simulink model "Single_Phase_Dual_converter_22UEE051"  (R2023b)
settings: Solver=VariableStepAuto  StartTime=0.0  StopTime=0.1  RelTol=1e-3
libraries: spsThyristorLib x8, spsVoltageMeasurementLib x5, spsSeriesRLCBranchLib x3, spsACVoltageSourceLib x2, spspowerguiLib x1
settings Model: Creator=prita  LastModifiedBy=SWARUP
settings DebuggingCC: UnconnectedInputMsg=warning  UnconnectedOutputMsg=warning  UnconnectedLineMsg=warning
settings ModelReferenceCC: EnableRefExpFcnMdlSchedulingChecks=on
settings RTWCC: DLArmComputeVersion=19.05

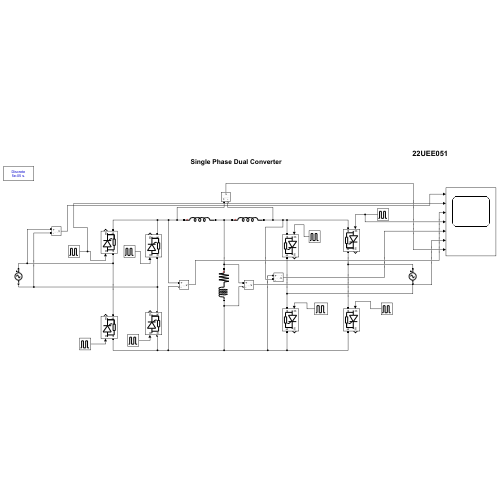
[thumbnail: Simulink's stored preview of the top-level diagram]
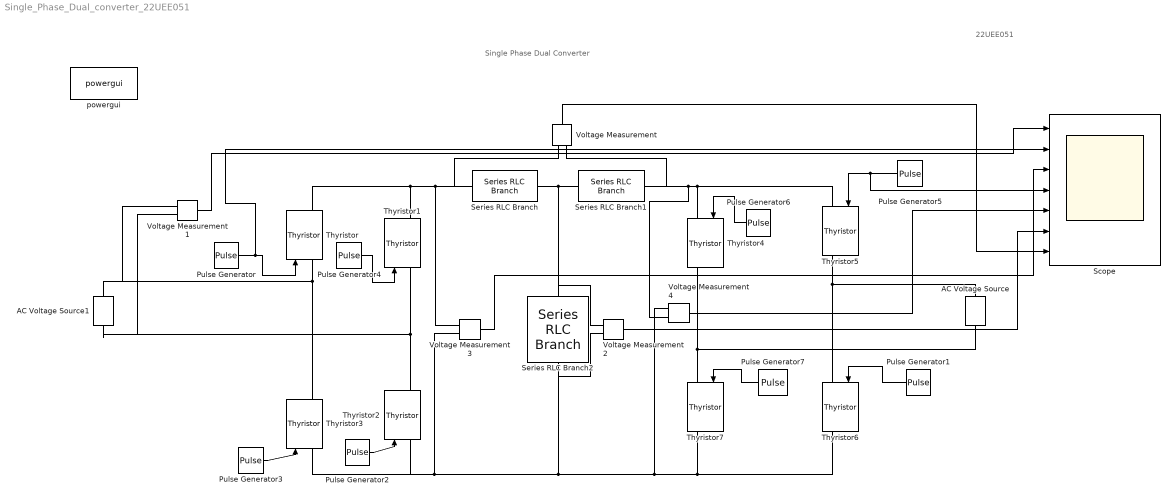
== system Single_Phase_Dual_converter_22UEE051 ==
  note: 22UEE051
  note: Single Phase Dual Converter
  AC Voltage Source : spsACVoltageSourceLib/AC Voltage Source  Amplitude=230  Phase=0  Frequency=50  SampleTime=0  Measurements=None  BusType=swing  Pref=10e3  Qref=0  Qmin=-inf  Qmax=+inf
  AC Voltage Source1 : spsACVoltageSourceLib/AC Voltage Source  Amplitude=230  Phase=0  Frequency=50  SampleTime=0  Measurements=None  BusType=swing  Pref=10e3  Qref=0  Qmin=-inf  Qmax=+inf
  Pulse Generator{,2..4} (4 alike) : DiscretePulseGenerator  PulseType=Time based  Amplitude=5  Period=0.01  PulseWidth=5  PhaseDelay=(0.02/360)*30
  Pulse Generator{1,5..7} (4 alike) : DiscretePulseGenerator  PulseType=Time based  Amplitude=5  Period=0.01  PulseWidth=5  PhaseDelay=(0.02/360)*150
  Scope : Scope  NumInputPorts=7
  Series RLC Branch : spsSeriesRLCBranchLib/Series RLC Branch  LConnTagsString=__new0  RConnTagsString=__new0  BranchType=L  Resistance=1  Inductance=0.5e-3  SetiL0=off  InitialCurrent=0  Capacitance=1e-6  Setx0=off  InitialVoltage=0  Measurements=None
  Series RLC Branch1 : spsSeriesRLCBranchLib/Series RLC Branch  LConnTagsString=__new0  RConnTagsString=__new0  BranchType=L  Resistance=1  Inductance=0.5e-3  SetiL0=off  InitialCurrent=0  Capacitance=1e-6  Setx0=off  InitialVoltage=0  Measurements=None
  Series RLC Branch2 : spsSeriesRLCBranchLib/Series RLC Branch  LConnTagsString=__new0  RConnTagsString=__new0  BranchType=RL  Resistance=2.15  Inductance=4.65e-3  SetiL0=off  InitialCurrent=0  Capacitance=1e-6  Setx0=off  InitialVoltage=0  Measurements=None
  Thyristor{,1..7} (8 alike) : spsThyristorLib/Thyristor  Ron=0.001  Lon=0  Vf=0.8  IC=0  Rs=500  Cs=250e-9  Measurements=on
  Voltage Measurement{,1..4} (5 alike) : spsVoltageMeasurementLib/Voltage Measurement  PhasorSimulation=off  OutputType=Complex  PSBequivalent=0
  powergui : spspowerguiLib/powergui  Priority=1  SimulationMode=Discrete  SampleTime=50e-6  frequency=60  Iterations=50  frequencyindice=50  Pbase=100e6  ErrMax=1e-4  UnitsV=kV  UnitsW=MW  buscounter=0  FunctionMessages=off  echomessages=off  EnableUseOfTLC=off  CurrentSourceSwitches=off  DisableSnubberDevices=off  DisableRonSwitches=off  DisableVfSwitches=off  DisplayEquations=off  AutomaticDiscreteSolvers=off  SolverType=Tustin/Backward Euler (TBE)  Interpol=off  ExternalGateDelay=off  methode=off  Ts=100  x0status=blocks  SPID=on  SwTol=0  HookPort=off  NonlinearTolerance=1e-4  nMaxIteration=100  ContinueOnMaxIteration=off  RestoreLinks=warning  ResistiveCurrentMeasurement=off  Frange=[0:2:500]  Ylog=off  Xlog=on  ShowGrid=off  save=off  variable=ZData  structure=0  ZoomFFT=off  StartTime=0.0  cycles=1  DisplayStyle=1  fundamental=60  FreqAxis=off  MaxFrequency=1000  frequencyindicesteady=1  RmsSteady=1  display=off
  wires:
  Pulse Generator5/1 -> Thyristor5/1, Scope/4
  Pulse Generator6/1 -> Thyristor4/1
  Pulse Generator7/1 -> Thyristor7/1
  Pulse Generator1/1 -> Thyristor6/1
  Pulse Generator4/1 -> Thyristor1/1
  Pulse Generator/1 -> Scope/2, Thyristor/1
  Pulse Generator3/1 -> Thyristor3/1
  Pulse Generator2/1 -> Thyristor2/1
  Voltage Measurement1/1 -> Scope/1
  Voltage Measurement3/1 -> Scope/3
  Voltage Measurement4/1 -> Scope/5
  Voltage Measurement2/1 -> Scope/6
  Voltage Measurement/1 -> Scope/7
  connections:
  Thyristor3/RConn1 -- Voltage Measurement1/LConn1 -- AC Voltage Source1/RConn1 -- Thyristor/LConn1
  Thyristor/RConn1 -- Voltage Measurement3/LConn1 -- Voltage Measurement/LConn1 -- Series RLC Branch/LConn1 -- Thyristor1/RConn1
  Thyristor2/RConn1 -- Voltage Measurement1/LConn2 -- AC Voltage Source1/LConn1 -- Thyristor1/LConn1
  Thyristor6/LConn1 -- AC Voltage Source/RConn1 -- Thyristor5/RConn1
  Thyristor7/LConn1 -- AC Voltage Source/LConn1 -- Thyristor4/RConn1
  Thyristor4/LConn1 -- Voltage Measurement4/LConn2 -- Voltage Measurement/LConn2 -- Series RLC Branch1/RConn1 -- Thyristor5/LConn1
  Thyristor7/RConn1 -- Voltage Measurement4/LConn1 -- Voltage Measurement3/LConn2 -- Thyristor2/LConn1 -- Thyristor3/LConn1 -- Series RLC Branch2/RConn1 -- Voltage Measurement2/LConn2 -- Thyristor6/RConn1
  Series RLC Branch1/LConn1 -- Series RLC Branch2/LConn1 -- Voltage Measurement2/LConn1 -- Series RLC Branch/RConn1
